simulink model "HojadeRecursos"  (R2016a)
settings: Solver=VariableStepAuto  StartTime=0.0  StopTime=10.0  RelTol=1e-3
libraries: commutil2 x6, commsrccod2 x4, commsynccomp2 x2, commcnvcod2 x2, commsink2 x2, sldrtlib x1, commchan3 x1
settings Model: Creator=Glynis  LastModifiedBy=Glynis

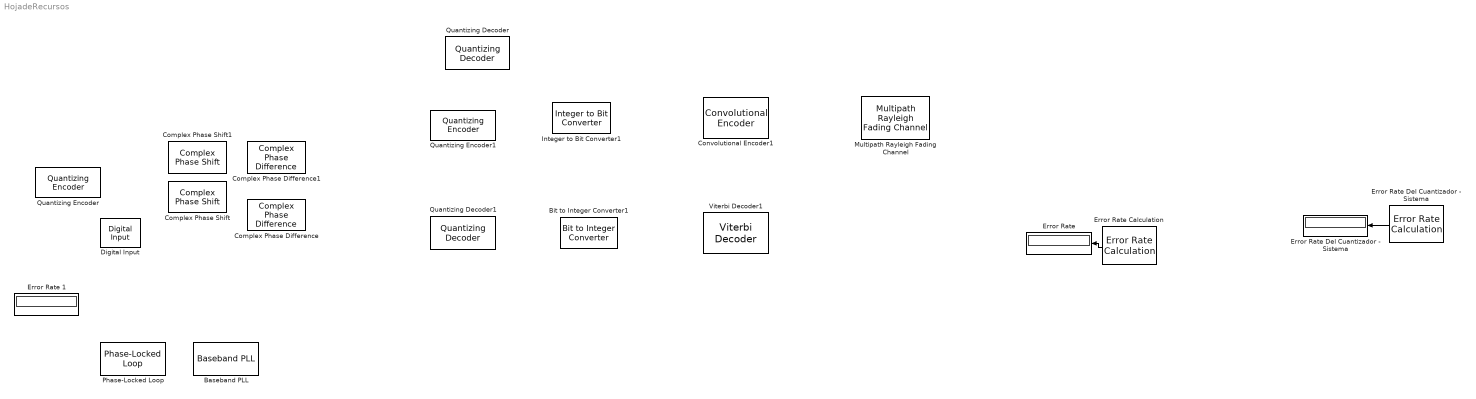
== system HojadeRecursos ==
  Baseband PLL : commsynccomp2/Baseband PLL  Fn="[3.0002  0  40002]"  Fd="[1   67.46   2270.9   40002]"  Kvco=1
  Bit to Integer Converter1 : commutil2/Bit to Integer Converter  nbits=3  bitOrder=MSB first  signedOutputValues=Unsigned  outDtype=Inherit via internal rule  outDtypeSigned=Inherit via internal rule
  Complex Phase Difference : commutil2/Complex Phase Difference
  Complex Phase Difference1 : commutil2/Complex Phase Difference
  Complex Phase Shift : commutil2/Complex Phase Shift
  Complex Phase Shift1 : commutil2/Complex Phase Shift
  Convolutional Encoder1 : commcnvcod2/Convolutional Encoder  trellis=poly2trellis(7, [171 133])  opMode=Continuous  DelayedResetAction=on  hasIniStPort=off  hasFinStPort=off  usePuncVector=off  punctureVector=[1; 1; 0; 1; 0; 1]  reset=Unused parameter value
  Digital Input : sldrtlib/Digital Input  SampleTime=0.1  MaxMissedTicks=10  ShowMissedTicks=off  YieldWhenWaiting=off  DrvAddress=0  DrvOptions=0  Channels=1  BitMode=1  DataType=1
  "Error Rate " : Display
  Error Rate 1 : Display
  Error Rate Calculation : commsink2/Error Rate Calculation  N=0  st_delay=0  cp_mode=Entire frame  subframe=[]  PMode=Port  WsName=ErrorVec  RsMode2=off  stop=off  numErr=100  maxBits=1e6
  "Error Rate Del Cuantizador - Sistema " : Display
  "Error Rate Del Cuantizador - Sistema " : commsink2/Error Rate Calculation  N=0  st_delay=0  cp_mode=Entire frame  subframe=[]  PMode=Port  WsName=ErrorVec  RsMode2=off  stop=off  numErr=100  maxBits=1e6
  Integer to Bit Converter1 : commutil2/Integer to Bit Converter  nbits=3  signedInputValues=Unsigned  bitOrder=MSB first  outDtype=Inherit via internal rule
  Multipath Rayleigh Fading Channel : commchan3/Multipath Rayleigh Fading Channel  maxDopplerShift=40  spectrumType=Jakes  sigmaGaussian=1/sqrt(2)  coeffRounded=[1 -1.72 0.785]  freqMinMaxRJakes=[0 1]  freqMinMaxAJakes=[0 1]  sigmaGaussian1=1/sqrt(2)  sigmaGaussian2=1/sqrt(2)  centerFreqGaussian1=0.0  centerFreqGaussian2=0.0  gainGaussian1=0.5  gainGaussian2=0.5  coeffBell=9  dopplerSpectrum=doppler.jakes  pathDelays=[0 2e-6]  avgPathGaindB=[0 -3]  normalizePathGains=on  seed=73  enableProbe=0  openVisAtStart=off  outPathGains=off  outDelay=off
  Phase-Locked Loop : commsynccomp2/Phase-Locked Loop  Fn="[3.0002  0  40002]"  Fd="[1   67.46   2270.9   40002]"  Kvco=1  Fc=100  Ph=0  Ac=1
  Quantizing Decoder : commsrccod2/Quantizing Decoder  codebook=[-.825 -.5 0, .5 .825]  QuDType=double
  Quantizing Decoder1 : commsrccod2/Quantizing Decoder  codebook=[-.825 -.5 0, .5 .825]  QuDType=double
  Quantizing Encoder : commsrccod2/Quantizing Encoder  partition=[-.75 -.25 .25 .75]  codebook=[-.825 -.5 0 .5 .825]  idxDType=double
  Quantizing Encoder1 : commsrccod2/Quantizing Encoder  partition=[-.75 -.25 .25 .75]  codebook=[-.825 -.5 0 .5 .825]  idxDType=double
  Viterbi Decoder1 : commcnvcod2/Viterbi Decoder  trellis=poly2trellis(7, [171 133])  isPunctured=off  punctureVector=[1; 1; 0; 1; 0; 1]  erasures=off  dectype=Hard decision  nsdecb=4  runSigValErrCheck=off  tbdepth=34  opmode=Continuous  reset=off  delayedResetAction=on  smWordLength=16  outDataType=Smallest unsigned integer
  wires:
  ? -> Error Rate Calculation/1
  ? -> Error Rate Calculation/2
  Error Rate Calculation/1 -> "Error Rate "/1
  ? -> "Error Rate Del Cuantizador - Sistema "/1
  ? -> "Error Rate Del Cuantizador - Sistema "/2
  "Error Rate Del Cuantizador - Sistema "/1 -> "Error Rate Del Cuantizador - Sistema "/1
